simulink model "joystick"  (R2022b)
settings: Solver=FixedStepAuto  StartTime=0.0  StopTime=inf  RelTol=1e-3  EnableMultiTasking=on
model workspace (MAT data in the model file):
  SL_ROS_VariableLengthArrays_MaxSizes.CommonInfo.ArrayTruncateAction = 'EmitWarning'
  SL_ROS_VariableLengthArrays_MaxSizes.MsgTypeMap = containers.Map
  SL_ROS_VariableLengthArrays_MaxSizes.MsgTypeMap.serialization.keys = {'sensor_msgs/Image'}
  SL_ROS_VariableLengthArrays_MaxSizes.MsgTypeMap.serialization.values{1}(1).PropertyName = 'Encoding'
  SL_ROS_VariableLengthArrays_MaxSizes.MsgTypeMap.serialization.values{1}(1).DataType = 'uint8'
  SL_ROS_VariableLengthArrays_MaxSizes.MsgTypeMap.serialization.values{1}(1).MaxLength = 5
  SL_ROS_VariableLengthArrays_MaxSizes.MsgTypeMap.serialization.values{1}(2).PropertyName = 'Data'
  SL_ROS_VariableLengthArrays_MaxSizes.MsgTypeMap.serialization.values{1}(2).DataType = 'uint8'
  SL_ROS_VariableLengthArrays_MaxSizes.MsgTypeMap.serialization.values{1}(2).MaxLength = 19200
  SL_ROS_VariableLengthArrays_MaxSizes.MsgTypeMap.serialization.uniformity = 0
  SL_ROS_VariableLengthArrays_MaxSizes.MsgTypeMap.serialization.keyType = 'char'
  SL_ROS_VariableLengthArrays_MaxSizes.MsgTypeMap.serialization.valueType = 'any'
settings Model: SimulationMode=external  ExtModeEnableFloating=off  Creator=The MathWorks, Inc.  LastModifiedBy=ebene
settings SolverCC: AlgebraicLoopSolver=TrustRegion  PositivePriorityOrder=on
settings DataIOCC: SaveFormat=Array  ReturnWorkspaceOutputs=off
settings OptimizationCC: EnhancedBackFolding=on  PassReuseOutputArgsThreshold=0  MaxStackSize=64  OptimizeBlockOrder=speed  DifferentSizesBufferReuse=on  OptimizationCustomize=off
settings DebuggingCC: SolverPrmCheckMsg=warning  ParameterTunabilityLossMsg=error  UnconnectedInputMsg=warning  UnconnectedOutputMsg=warning  UnconnectedLineMsg=warning  AllowSymbolicDim=off  SFUnexpectedBacktrackingDiag=warning  SFNoUnconditionalDefaultTransitionDiag=warning  SFMachineParentedDataDiag=warning  ArithmeticOperatorsInVariantConditions=warning
settings HardwareCC: ProdBitPerPointer=32  ProdBitPerSizeT=32  ProdBitPerPtrDiffT=32  ProdLargestAtomicInteger=Long  ProdLargestAtomicFloat=Double  ProdWordSize=32  ProdLongLongMode=on  ProdHWDeviceType=ARM Compatible->ARM Cortex
settings ModelReferenceCC: EnableRefExpFcnMdlSchedulingChecks=on  PropagateSignalLabelsOutOfModel=off
settings SFSimCC: SimUseLocalCustomCode=off  CustomCodeUndefinedFunction=UseInterfaceOnly
settings RTWCC: Description=Embedded Coder  SystemTargetFile=ert.tlc  HardwareBoard=Raspberry Pi  TLCOptions="-aInlineSetEventsForThisBaseRateFcn=TLC_FALSE -aSuppressMultiTaskScheduler=TLC_FALSE  -aRateBasedStepFcn=0"  TemplateMakefile=ert_default_tmf  RTWUseLocalCustomCode=off  Toolchain=GNU GCC Embedded Linux  BuildConfiguration=Faster Runs  DLArmComputeVersion=19.05
settings CodeAppCC: ForceParamTrailComments=on  OperatorAnnotations=on
settings ERTTargetCC: ERTCustomFileBanners=off  SupportContinuousTime=on  SupportNonInlinedSFcns=on  RemoveResetFunc=off  SupportVariableSizeSignals=on  ModelStepFunctionPrototypeControlCompliant=off  ExtModeTransport=2  ExtModeStaticAlloc=on  ExtModeMexFile=ext_xcp  ExtModeIntrfLevel=Level2 - Open
settings ConfigComp: CovMetricSettings=dw  CovSaveCumulativeToWorkspaceVar=on  CovSaveSingleToWorkspaceVar=on  CovExternalEMLEnable=off  CovSFcnEnable=off

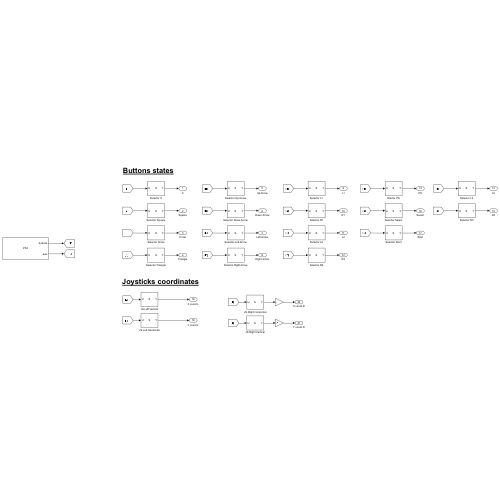
[thumbnail: Simulink's stored preview of the top-level diagram]
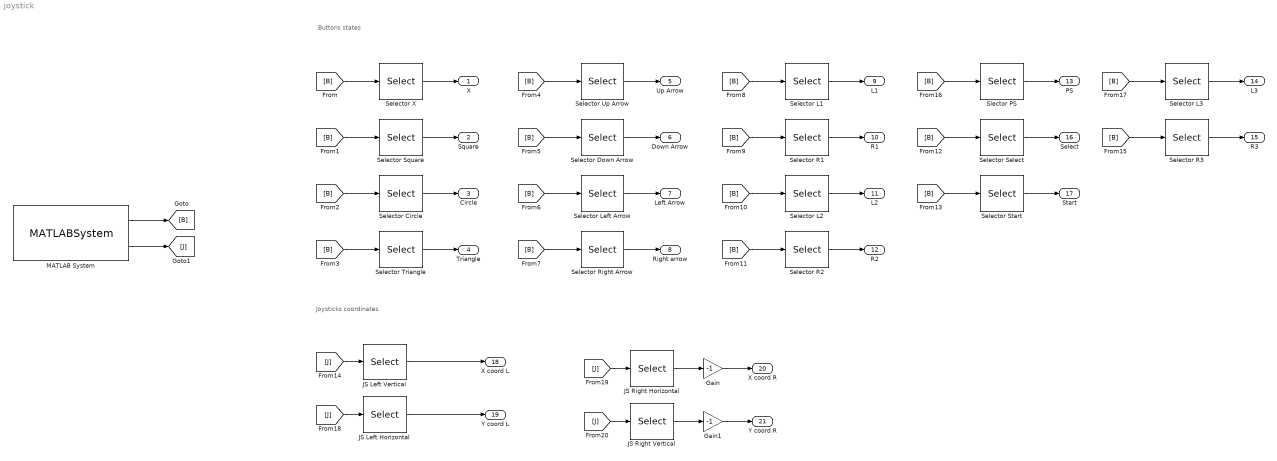
== system joystick ==
  note: Joysticks coordinates
  note: Buttons states
  Gain : Gain  Gain=-1
  Gain1 : Gain  Gain=-1
  JS Left Horizontal : Selector  NumberOfDimensions=2  IndexMode=Zero-based  InputPortWidth=3  IndexOptions=Index vector (dialog),Index vector (dialog)  Indices=0,0  OutputSizes=1,1
  JS Left Vertical : Selector  NumberOfDimensions=2  IndexMode=Zero-based  InputPortWidth=3  IndexOptions=Index vector (dialog),Index vector (dialog)  Indices=0,1  OutputSizes=1,1
  JS Right Horizontal : Selector  NumberOfDimensions=2  IndexMode=Zero-based  InputPortWidth=3  IndexOptions=Index vector (dialog),Index vector (dialog)  Indices=0,3  OutputSizes=1,1
  JS Right Vertical : Selector  NumberOfDimensions=2  IndexMode=Zero-based  InputPortWidth=3  IndexOptions=Index vector (dialog),Index vector (dialog)  Indices=0,4  OutputSizes=1,1
  MATLAB System : MATLABSystem  System=PS3  SampleTime=0.01
      mask Type: PS3
      mask Display:
      | disp('PS3');
      | port_label('output',1,'buttons');
      | port_label('output',2,'axis');
  Selector Circle : Selector  NumberOfDimensions=2  IndexMode=Zero-based  InputPortWidth=3  IndexOptions=Index vector (dialog),Index vector (dialog)  Indices=0,1  OutputSizes=1,1
  Selector Down Arrow : Selector  NumberOfDimensions=2  IndexMode=Zero-based  InputPortWidth=3  IndexOptions=Index vector (dialog),Index vector (dialog)  Indices=0,14  OutputSizes=1,1
  Selector L1 : Selector  NumberOfDimensions=2  IndexMode=Zero-based  InputPortWidth=3  IndexOptions=Index vector (dialog),Index vector (dialog)  Indices=0,4  OutputSizes=1,1
  Selector L2 : Selector  NumberOfDimensions=2  IndexMode=Zero-based  InputPortWidth=3  IndexOptions=Index vector (dialog),Index vector (dialog)  Indices=0,6  OutputSizes=1,1
  Selector L3 : Selector  NumberOfDimensions=2  IndexMode=Zero-based  InputPortWidth=3  IndexOptions=Index vector (dialog),Index vector (dialog)  Indices=0,11  OutputSizes=1,1
  Selector Left Arrow : Selector  NumberOfDimensions=2  IndexMode=Zero-based  InputPortWidth=3  IndexOptions=Index vector (dialog),Index vector (dialog)  Indices=0,15  OutputSizes=1,1
  Selector R1 : Selector  NumberOfDimensions=2  IndexMode=Zero-based  InputPortWidth=3  IndexOptions=Index vector (dialog),Index vector (dialog)  Indices=0,5  OutputSizes=1,1
  Selector R2 : Selector  NumberOfDimensions=2  IndexMode=Zero-based  InputPortWidth=3  IndexOptions=Index vector (dialog),Index vector (dialog)  Indices=0,7  OutputSizes=1,1
  Selector R3 : Selector  NumberOfDimensions=2  IndexMode=Zero-based  InputPortWidth=3  IndexOptions=Index vector (dialog),Index vector (dialog)  Indices=0,12  OutputSizes=1,1
  Selector Right Arrow : Selector  NumberOfDimensions=2  IndexMode=Zero-based  InputPortWidth=3  IndexOptions=Index vector (dialog),Index vector (dialog)  Indices=0,16  OutputSizes=1,1
  Selector Select : Selector  NumberOfDimensions=2  IndexMode=Zero-based  InputPortWidth=3  IndexOptions=Index vector (dialog),Index vector (dialog)  Indices=0,8  OutputSizes=1,1
  Selector Square : Selector  NumberOfDimensions=2  IndexMode=Zero-based  InputPortWidth=3  IndexOptions=Index vector (dialog),Index vector (dialog)  Indices=0,3  OutputSizes=1,1
  Selector Start : Selector  NumberOfDimensions=2  IndexMode=Zero-based  InputPortWidth=3  IndexOptions=Index vector (dialog),Index vector (dialog)  Indices=0,9  OutputSizes=1,1
  Selector Triangle : Selector  NumberOfDimensions=2  IndexMode=Zero-based  InputPortWidth=3  IndexOptions=Index vector (dialog),Index vector (dialog)  Indices=0,2  OutputSizes=1,1
  Selector Up Arrow : Selector  NumberOfDimensions=2  IndexMode=Zero-based  InputPortWidth=3  IndexOptions=Index vector (dialog),Index vector (dialog)  Indices=0,13  OutputSizes=1,1
  Selector X : Selector  NumberOfDimensions=2  IndexMode=Zero-based  InputPortWidth=3  IndexOptions=Index vector (dialog),Index vector (dialog)  Indices=0,0  OutputSizes=1,1
  Slector PS : Selector  NumberOfDimensions=2  IndexMode=Zero-based  InputPortWidth=3  IndexOptions=Index vector (dialog),Index vector (dialog)  Indices=0,10  OutputSizes=1,1
  X : Outport
  Square : Outport  Port=2
  Circle : Outport  Port=3
  Triangle : Outport  Port=4
  Up Arrow : Outport  Port=5
  Down Arrow : Outport  Port=6
  Left Arrow : Outport  Port=7
  Right arrow : Outport  Port=8
  L1 : Outport  Port=9
  R1 : Outport  Port=10
  L2 : Outport  Port=11
  R2 : Outport  Port=12
  PS : Outport  Port=13
  L3 : Outport  Port=14
  R3 : Outport  Port=15
  Select : Outport  Port=16
  Start : Outport  Port=17
  X coord L : Outport  Port=18
  Y coord L : Outport  Port=19
  X coord R : Outport  Port=20
  Y coord R : Outport  Port=21
  wires:
  Selector X/1 -> X/1
  MATLAB System/1 -> [B]
  [B] -> Selector X/1
  Selector Square/1 -> Square/1
  Selector Circle/1 -> Circle/1
  Selector Triangle/1 -> Triangle/1
  [B] -> Selector Square/1
  [B] -> Selector Circle/1
  [B] -> Selector Triangle/1
  Selector Up Arrow/1 -> Up Arrow/1
  Selector Down Arrow/1 -> Down Arrow/1
  Selector Left Arrow/1 -> Left Arrow/1
  Selector Right Arrow/1 -> Right arrow/1
  [B] -> Selector Up Arrow/1
  [B] -> Selector Right Arrow/1
  [B] -> Selector Left Arrow/1
  [B] -> Selector Down Arrow/1
  [B] -> Selector L2/1
  Selector R1/1 -> R1/1
  Selector L1/1 -> L1/1
  [B] -> Selector R1/1
  [B] -> Selector R2/1
  [B] -> Selector L1/1
  Selector R2/1 -> R2/1
  Selector L2/1 -> L2/1
  Selector L3/1 -> L3/1
  [B] -> Selector L3/1
  [B] -> Slector PS/1
  Slector PS/1 -> PS/1
  [B] -> Selector R3/1
  Selector R3/1 -> R3/1
  Selector Select/1 -> Select/1
  [B] -> Selector Select/1
  Selector Start/1 -> Start/1
  [B] -> Selector Start/1
  JS Left Horizontal/1 -> Y coord L/1
  JS Left Vertical/1 -> X coord L/1
  MATLAB System/2 -> [J]
  [J] -> JS Left Vertical/1
  [J] -> JS Left Horizontal/1
  [J] -> JS Right Horizontal/1
  [J] -> JS Right Vertical/1
  JS Right Horizontal/1 -> Gain/1
  Gain/1 -> X coord R/1
  Gain1/1 -> Y coord R/1
  JS Right Vertical/1 -> Gain1/1
